simulink model "problem7"  (R2023a)
settings: Solver=VariableStepAuto  StartTime=0.0  StopTime=6  RelTol=1e-10
settings Model: Creator=mcconncm  LastModifiedBy=mcconncm

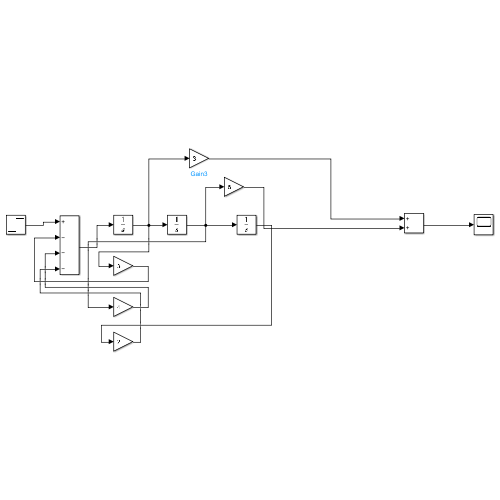
[thumbnail: Simulink's stored preview of the top-level diagram]
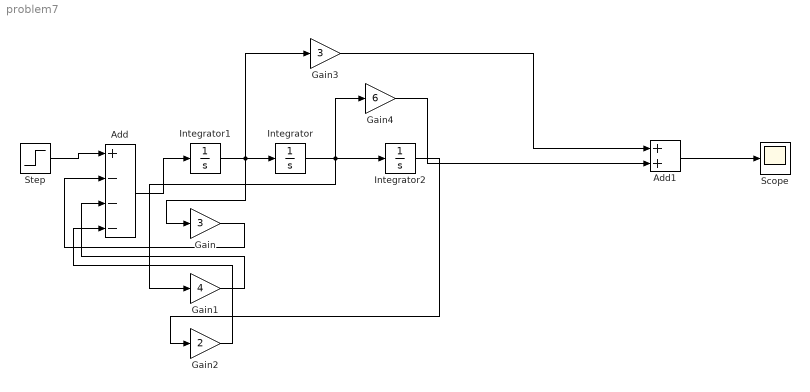
== system problem7 ==
  Add : Sum  Inputs=+---
  Add1 : Sum
  Gain : Gain  Gain=3
  Gain1 : Gain  Gain=4
  Gain2 : Gain  Gain=2
  Gain3 : Gain  Gain=3
  Gain4 : Gain  Gain=6
  Integrator : Integrator
  Integrator1 : Integrator
  Integrator2 : Integrator
  Scope : Scope
  Step : Step  Time=0  SampleTime=0
  wires:
  Integrator1/1 -> Gain3/1, Gain/1, Integrator/1
  Integrator/1 -> Gain4/1, Gain1/1, Integrator2/1
  Step/1 -> Add/1
  Add/1 -> Integrator1/1
  Gain1/1 -> Add/3
  Gain/1 -> Add/2
  Gain2/1 -> Add/4
  Integrator2/1 -> Gain2/1
  Gain3/1 -> Add1/1
  Gain4/1 -> Add1/2
  Add1/1 -> Scope/1
